simulink model "onlab_lidar1"  (R2023b)
settings: Solver=FixedStepDiscrete  StartTime=0.0  StopTime=15  RelTol=1e-3
model workspace (MAT data in the model file):
  firstWarning = 1
  originalScenarioChecksum = 'B723F0CC9A03C13659EA1EEED9D3BEC3'
libraries: drivingscenarioandsensors x2
settings Model: Creator=Mate  LastModifiedBy=Mate

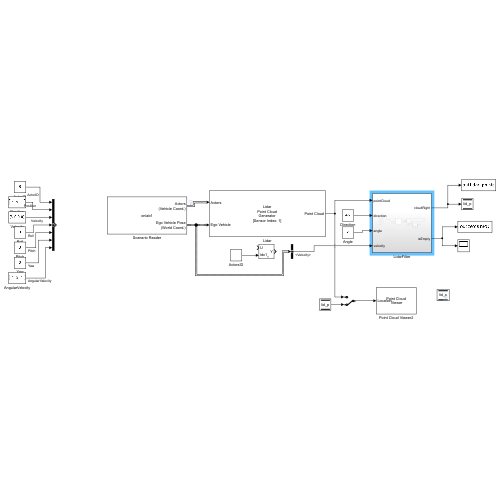
[thumbnail: Simulink's stored preview of the top-level diagram]
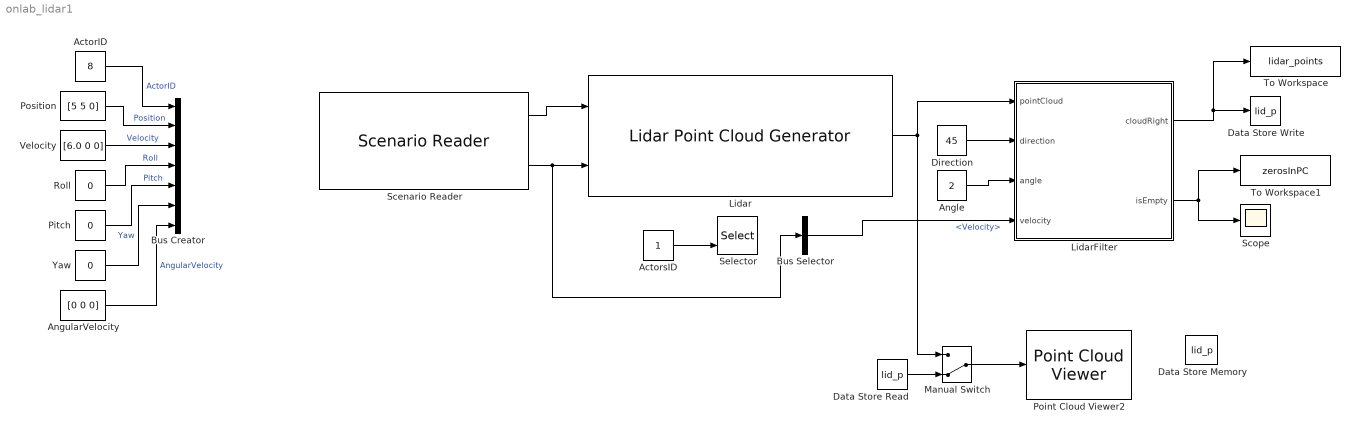
== system onlab_lidar1 ==
  ActorID : Constant  Value=8
  ActorsID : Constant
  Angle : Constant  Value=2
  AngularVelocity : Constant  Value=[0 0 0]  VectorParams1D=off
  Bus Creator : BusCreator  Inputs=7  OutDataTypeStr=Bus: myActorBus  NonVirtualBus=on
  Bus Selector : BusSelector  OutputSignals=Velocity
  Data Store Memory : DataStoreMemory  DataStoreName=lid_p  WriteAfterWriteMsg=warning  InitialValue=zeros(20,180,3)  VectorParams1D=off  ShowAdditionalParam=off  OutDataTypeStr=double
  Data Store Read : DataStoreRead  DataStoreName=lid_p  IndexOptions=Index vector (dialog)  Indices=1  OutputSizes=1
  Data Store Write : DataStoreWrite  DataStoreName=lid_p  IndexOptions=Index vector (dialog)  Indices=1  OutputSizes=1
  Direction : Constant  Value=45
  Lidar : drivingscenarioandsensors/Lidar Point Cloud Generator  SensorIndex=1  UpdateInterval=0.1  SensorLocation=[0.95 0]  Height=1.6  Yaw=0  Pitch=0  Roll=0  DetectionCoordinates=Sensor Cartesian  HasEgoVehicle=on  EgoVehicleActorID=8  HasRoadsInputPort=on  ActorProfilesSource=From Scenario Reader block  ActorProfilesVariableName=actor_profiles  MaxRange=120  RangeAccuracy=0.005  AzimuthResolution=2  ElevationResolution=2  AzimuthLimits=[-180 180]  ElevationLimits=[-20 20]  HasNoise=off
  LidarFilter : Subsystem
  Manual Switch : ManualSwitch  CurrentSetting=0
  Pitch : Constant  Value=0
  Point Cloud Viewer2 : PointCloudViewer  FigPos=[-1919 1038 1920 964.8]
  Position : Constant  Value=[5 5 0]  VectorParams1D=off
  Roll : Constant  Value=0
  Scenario Reader : drivingscenarioandsensors/Scenario Reader  ScenarioSource=From file  ScenarioFileName=C:\Users\Mate\Documents\MATLAB\MScOnlab1\onlab1.mat  ScenarioVariableName=scenario  OutputCoordinateSystem=Vehicle coordinates  EgoVehicleSource=Scenario  EgoVehicleActorID=1  OrientVehiclesOnRoad=on  OutputEgoVehiclePose=on  OutputEgoVehicleState=off  SampleTime=0.1  LaneBoundaryOutput=None  LaneBoundaryDistance=0:0.5:9.5  LaneBoundaryLocation=Center of lane markings  BusNameSource=Auto  BusName=BusActors  BusNumActorsSource=Scenario  BusNumActors=100  BusName2Source=Auto  BusName2=BusLaneBoundaries  BusNumLaneBoundariesSource=Scenario  BusNumLaneBoundaries=10  BusName3Source=Auto  BusName3=BusEgoActor  BusName4Source=Auto  BusName4=BusEgoState  ShowCoordinateLabels=on  SimulateUsing=Interpreted execution
  Scope : Scope
  Selector : Selector  InputPortWidth=3  IndexOptions=Index vector (port)  Indices=[1 3]  OutputSizes=1
  To Workspace : ToWorkspace  VariableName=lidar_points  SampleTime=-1
  To Workspace1 : ToWorkspace  VariableName=zerosInPC  SaveFormat=Timeseries  SampleTime=-1
  Velocity : Constant  Value=[6.0 0 0]  VectorParams1D=off
  Yaw : Constant  Value=0
  wires:
  Scenario Reader/1 -> Lidar/1
  Data Store Read/1 -> Manual Switch/2
  ActorID/1 -> Bus Creator/1  "ActorID"
  Position/1 -> Bus Creator/2  "Position"
  Velocity/1 -> Bus Creator/3  "Velocity"
  Roll/1 -> Bus Creator/4  "Roll"
  Pitch/1 -> Bus Creator/5  "Pitch"
  Yaw/1 -> Bus Creator/6  "Yaw"
  AngularVelocity/1 -> Bus Creator/7  "AngularVelocity"
  Lidar/1 -> LidarFilter/1(pointCloud), Manual Switch/1
  Scenario Reader/2 -> Bus Selector/1, Lidar/2
  Manual Switch/1 -> Point Cloud Viewer2/1
  LidarFilter/2(isEmpty) -> To Workspace1/1, Scope/1
  LidarFilter/1(cloudRight) -> To Workspace/1, Data Store Write/1
  Direction/1 -> LidarFilter/2(direction)
  Angle/1 -> LidarFilter/3(angle)
  ActorsID/1 -> Selector/2
  Bus Selector/1 -> LidarFilter/4(velocity)  "<Velocity>"

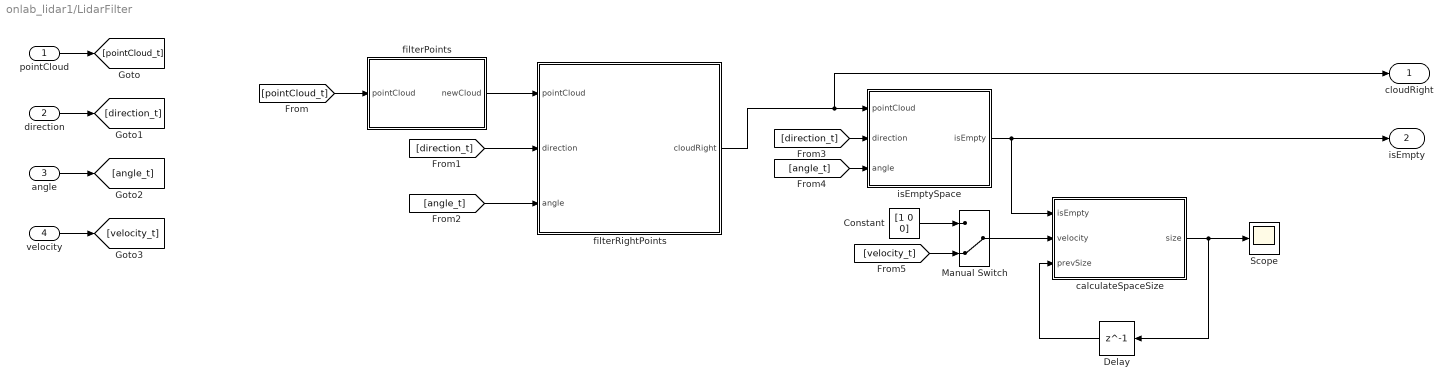
== system onlab_lidar1/LidarFilter ==
  pointCloud : Inport
  direction : Inport  Port=2
  angle : Inport  Port=3
  velocity : Inport  Port=4
  Constant : Constant  Value=[1 0 0]
  Delay : Delay  DelayLength=1
  Manual Switch : ManualSwitch  CurrentSetting=0
  Scope : Scope
  calculateSpaceSize : MATLAB Function  TreatAsAtomicUnit=on
  filterPoints : MATLAB Function  TreatAsAtomicUnit=on
  filterRightPoints : MATLAB Function  TreatAsAtomicUnit=on
  isEmptySpace : MATLAB Function  TreatAsAtomicUnit=on
  cloudRight : Outport
  isEmpty : Outport  Port=2
  wires:
  filterPoints/1(newCloud) -> filterRightPoints/1(pointCloud)
  filterRightPoints/1(cloudRight) -> cloudRight/1, isEmptySpace/1(pointCloud)
  pointCloud/1 -> [pointCloud_t]
  [pointCloud_t] -> filterPoints/1(pointCloud)
  direction/1 -> [direction_t]
  angle/1 -> [angle_t]
  [direction_t] -> filterRightPoints/2(direction)
  [angle_t] -> filterRightPoints/3(angle)
  [direction_t] -> isEmptySpace/2(direction)
  [angle_t] -> isEmptySpace/3(angle)
  isEmptySpace/1(isEmpty) -> calculateSpaceSize/1(isEmpty), isEmpty/1
  calculateSpaceSize/1(size) -> Delay/1, Scope/1
  velocity/1 -> [velocity_t]
  Delay/1 -> calculateSpaceSize/3(prevSize)
  Manual Switch/1 -> calculateSpaceSize/2(velocity)
  Constant/1 -> Manual Switch/1
  [velocity_t] -> Manual Switch/2

== matlab function onlab_lidar1/LidarFilter/filterRightPoints ==
  data: pointCloud input; cloudRight output; direction input; angle input
function cloudRight = filterRightPoints(pointCloud, direction, angle)
    xCoord = 1;
    yCoord = 2;
    maxIdx = 180;
    cloud = zeros(20,maxIdx,3);

    for row=1:20
        % Ha leírja a teljes kört a direction és az angle, akkor visszadja
        % a teljes ponthalmazt
        if (direction+angle) > maxIdx && (direction-angle) < 0
            cloud = pointCloud;
        else
            % Ha nem lóg át a maxIdx|1 határon a lekért ponthalmaz, akkor
            % ezeket a pontokat átmásolja
            if direction > angle && (direction + angle) < maxIdx
                for col = direction-angle:direction+angle
                    for idx=xCoord:yCoord
                        cloud(row,col,idx) = pointCloud(row,col,idx);
                    end
                end
            % Ha átlóg a kért pontfelhő a maxIdx|1 határon, akkor két
            % részre osztva másolja át
            else
                for col = 1:mod((direction+angle),maxIdx)
                    for idx=xCoord:yCoord
                        cloud(row,col,idx) = pointCloud(row,col,idx);
                    end
                end
                for col = maxIdx:mod((direction-angle+maxIdx),maxIdx)
                    for idx=xCoord:yCoord
                        cloud(row,col,idx) = pointCloud(row,col,idx);
                    end
                end
            end
        end
    end
    
cloudRight = cloud;

== matlab function onlab_lidar1/LidarFilter/filterPoints ==
  data: pointCloud input; newCloud output
function newCloud = filterPoints(pointCloud)
    cloud = zeros(20,180,3);
    for row=1:20
        for col=1:180
            if pointCloud(row,col,3) > -1.55 && pointCloud(row,col,3) < 1.5 ...
                   && abs(pointCloud(row,col,2)) > 0.9
                for coord=1:2
                    cloud(row,col,coord) = pointCloud(row,col,coord);
                end
                cloud(row,col,3) = 0;
            end
        end
    end
newCloud = cloud;

== matlab function onlab_lidar1/LidarFilter/isEmptySpace ==
  data: pointCloud input; isEmpty output; direction input; angle input
function isEmpty = cntEmptyRows(pointCloud, direction, angle)
    maxIdx = 180;
    sumZeros = 0;
    % Count zeros:
    if (direction+angle) > maxIdx && (direction-angle) < 0
        % do nothing
    else
        if direction > angle && (direction + angle) < maxIdx
            for col = direction-angle:direction+angle
                zerosInRow = 0;
                for row = 1:20
                    if pointCloud(row,col,1) == 0 && pointCloud(row,col,2) == 0
                        zerosInRow = zerosInRow + 1;
                    end
                end
                if zerosInRow == 20
                    sumZeros = sumZeros + 1;
                end
            end
        % Ha átlóg a kért pontfelhő a maxIdx|1 határon, akkor két
        % részre osztva vizsgálja
        else
            for col = 1:mod((direction+angle),maxIdx)
                zerosInRow = 0;
                for row = 1:20
                    if pointCloud(row,col,1) == 0 && pointCloud(row,col,2) == 0
                        zerosInRow = zerosInRow + 1;
                    end
                end
                if zerosInRow == 20
                    sumZeros = sumZeros + 1;
                end
            end
            for col = maxIdx:mod((direction-angle+maxIdx),maxIdx)
                zerosInRow = 0;
                for row = 1:20
                    if pointCloud(row,col,1) == 0 && pointCloud(row,col,2) == 0
                        zerosInRow = zerosInRow + 1;
                    end
                end
                if zerosInRow == 20
                    sumZeros = sumZeros + 1;
                end
            end
        end
    end
    if sumZeros == (2*angle+1)
        isEmpty = true;
    else
        isEmpty = false;
    end
    
% isEmpty = sumZeros;

== matlab function onlab_lidar1/LidarFilter/calculateSpaceSize ==
  data: isEmpty input; size output; velocity input; prevSize input
function size = calculateSpaceSize(isEmpty, velocity, prevSize)
    T = 0.1;
    if isEmpty
        size = prevSize + T * norm(velocity);
    else
        size = 0;
    end
